simulink subsystem "tractive"  (R2023b)
settings: Solver=VariableStepAuto  StartTime=0.0  StopTime=10.0  RelTol=1e-3
libraries: Raptor_lib x11
settings Model: Creator=serga  LastModifiedBy=serga

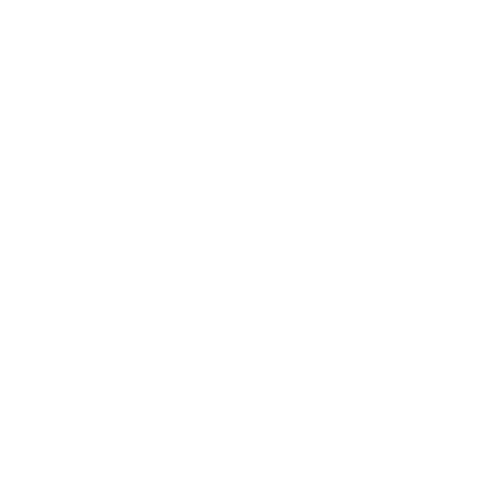
[thumbnail: Simulink's stored preview of the top-level diagram]
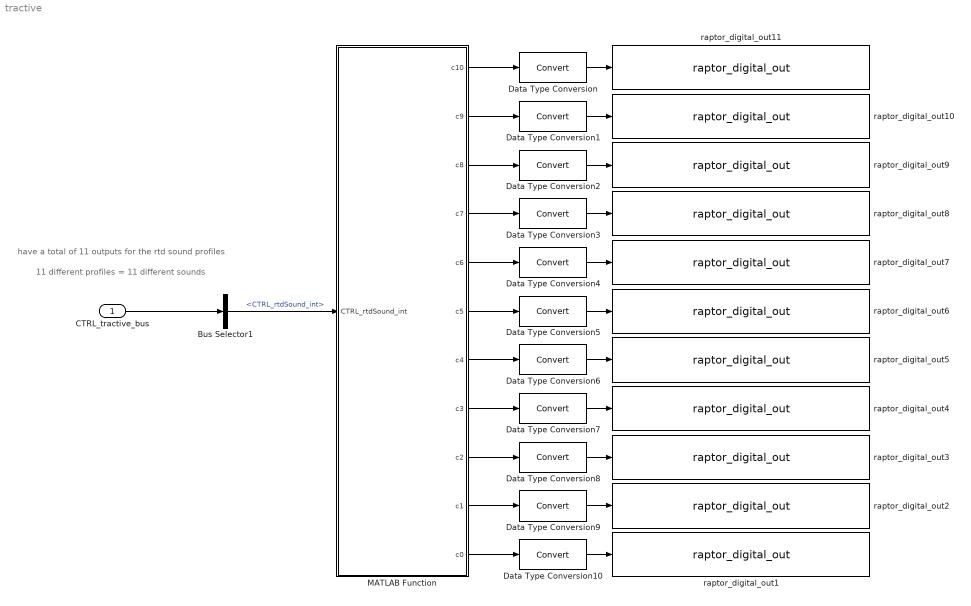
== system tractive ==
  note: 11 different profiles = 11 different sounds
  note: have a total of 11 outputs for the rtd sound profiles
  CTRL_tractive_bus : Inport
  Bus Selector1 : BusSelector  OutputSignals=CTRL_rtdSound_int
  Data Type Conversion{,1..10} (11 alike) : DataTypeConversion  SaturateOnIntegerOverflow=off  RndMeth=Floor
  MATLAB Function : MATLAB Function  TreatAsAtomicUnit=on
  raptor_digital_out1 : Raptor_lib/Input & Output/raptor_digital_out  resourceValues=OUTPUT1|OUTPUT2|OUTPUT3|OUTPUT4|OUTPUT5|OUTPUT6|OUTPUT7|OUTPUT8|OUTPUT9|OUTPUT10|OUTPUT11|OUTPUT12|OUTPUT21|OUTPUT22|OUTPUT23|OUTPUT24|OUTPUT25|OUTPUT26|OUTPUT27|OUTPUT28|OUTPUT29|OUTPUT30|OUTPUT31|OUTPUT32|OUTPUT33|OUTPUT34|OUTPUT35|OUTPUT36|OUTPUT37|OUTPUT38|OUTPUT39|OUTPUT40|OUTPUT41|OUTPUT42|OUTPUT43|OUTPUT44|OUTPUT45|OUTPUT46|OUTPUT47|OUTPUT48|OUTPUT49|POWER_HOLD|(None)  resource=OUTPUT4  driverTypeValues=Low Side  driverType=Low Side
      settings: SourceProductName=Raptor
  raptor_digital_out10 : Raptor_lib/Input & Output/raptor_digital_out  resourceValues=OUTPUT1|OUTPUT2|OUTPUT3|OUTPUT4|OUTPUT5|OUTPUT6|OUTPUT7|OUTPUT8|OUTPUT9|OUTPUT10|OUTPUT11|OUTPUT12|OUTPUT21|OUTPUT22|OUTPUT23|OUTPUT24|OUTPUT25|OUTPUT26|OUTPUT27|OUTPUT28|OUTPUT29|OUTPUT30|OUTPUT31|OUTPUT32|OUTPUT33|OUTPUT34|OUTPUT35|OUTPUT36|OUTPUT37|OUTPUT38|OUTPUT39|OUTPUT40|OUTPUT41|OUTPUT42|OUTPUT43|OUTPUT44|OUTPUT45|OUTPUT46|OUTPUT47|OUTPUT48|OUTPUT49|POWER_HOLD|(None)  resource=OUTPUT32  driverTypeValues=Low Side  driverType=Low Side
      settings: SourceProductName=Raptor
  raptor_digital_out11 : Raptor_lib/Input & Output/raptor_digital_out  resourceValues=OUTPUT1|OUTPUT2|OUTPUT3|OUTPUT4|OUTPUT5|OUTPUT6|OUTPUT7|OUTPUT8|OUTPUT9|OUTPUT10|OUTPUT11|OUTPUT12|OUTPUT21|OUTPUT22|OUTPUT23|OUTPUT24|OUTPUT25|OUTPUT26|OUTPUT27|OUTPUT28|OUTPUT29|OUTPUT30|OUTPUT31|OUTPUT32|OUTPUT33|OUTPUT34|OUTPUT35|OUTPUT36|OUTPUT37|OUTPUT38|OUTPUT39|OUTPUT40|OUTPUT41|OUTPUT42|OUTPUT43|OUTPUT44|OUTPUT45|OUTPUT46|OUTPUT47|OUTPUT48|OUTPUT49|POWER_HOLD|(None)  resource=OUTPUT35  driverTypeValues=Low Side  driverType=Low Side
      settings: SourceProductName=Raptor
  raptor_digital_out2 : Raptor_lib/Input & Output/raptor_digital_out  resourceValues=OUTPUT1|OUTPUT2|OUTPUT3|OUTPUT4|OUTPUT5|OUTPUT6|OUTPUT7|OUTPUT8|OUTPUT9|OUTPUT10|OUTPUT11|OUTPUT12|OUTPUT21|OUTPUT22|OUTPUT23|OUTPUT24|OUTPUT25|OUTPUT26|OUTPUT27|OUTPUT28|OUTPUT29|OUTPUT30|OUTPUT31|OUTPUT32|OUTPUT33|OUTPUT34|OUTPUT35|OUTPUT36|OUTPUT37|OUTPUT38|OUTPUT39|OUTPUT40|OUTPUT41|OUTPUT42|OUTPUT43|OUTPUT44|OUTPUT45|OUTPUT46|OUTPUT47|OUTPUT48|OUTPUT49|POWER_HOLD|(None)  resource=OUTPUT22  driverTypeValues=Low Side  driverType=Low Side
      settings: SourceProductName=Raptor
  raptor_digital_out3 : Raptor_lib/Input & Output/raptor_digital_out  resourceValues=OUTPUT1|OUTPUT2|OUTPUT3|OUTPUT4|OUTPUT5|OUTPUT6|OUTPUT7|OUTPUT8|OUTPUT9|OUTPUT10|OUTPUT11|OUTPUT12|OUTPUT21|OUTPUT22|OUTPUT23|OUTPUT24|OUTPUT25|OUTPUT26|OUTPUT27|OUTPUT28|OUTPUT29|OUTPUT30|OUTPUT31|OUTPUT32|OUTPUT33|OUTPUT34|OUTPUT35|OUTPUT36|OUTPUT37|OUTPUT38|OUTPUT39|OUTPUT40|OUTPUT41|OUTPUT42|OUTPUT43|OUTPUT44|OUTPUT45|OUTPUT46|OUTPUT47|OUTPUT48|OUTPUT49|POWER_HOLD|(None)  resource=OUTPUT24  driverTypeValues=Low Side  driverType=Low Side
      settings: SourceProductName=Raptor
  raptor_digital_out4 : Raptor_lib/Input & Output/raptor_digital_out  resourceValues=OUTPUT1|OUTPUT2|OUTPUT3|OUTPUT4|OUTPUT5|OUTPUT6|OUTPUT7|OUTPUT8|OUTPUT9|OUTPUT10|OUTPUT11|OUTPUT12|OUTPUT21|OUTPUT22|OUTPUT23|OUTPUT24|OUTPUT25|OUTPUT26|OUTPUT27|OUTPUT28|OUTPUT29|OUTPUT30|OUTPUT31|OUTPUT32|OUTPUT33|OUTPUT34|OUTPUT35|OUTPUT36|OUTPUT37|OUTPUT38|OUTPUT39|OUTPUT40|OUTPUT41|OUTPUT42|OUTPUT43|OUTPUT44|OUTPUT45|OUTPUT46|OUTPUT47|OUTPUT48|OUTPUT49|POWER_HOLD|(None)  resource=OUTPUT25  driverTypeValues=Low Side  driverType=Low Side
      settings: SourceProductName=Raptor
  raptor_digital_out5 : Raptor_lib/Input & Output/raptor_digital_out  resourceValues=OUTPUT1|OUTPUT2|OUTPUT3|OUTPUT4|OUTPUT5|OUTPUT6|OUTPUT7|OUTPUT8|OUTPUT9|OUTPUT10|OUTPUT11|OUTPUT12|OUTPUT21|OUTPUT22|OUTPUT23|OUTPUT24|OUTPUT25|OUTPUT26|OUTPUT27|OUTPUT28|OUTPUT29|OUTPUT30|OUTPUT31|OUTPUT32|OUTPUT33|OUTPUT34|OUTPUT35|OUTPUT36|OUTPUT37|OUTPUT38|OUTPUT39|OUTPUT40|OUTPUT41|OUTPUT42|OUTPUT43|OUTPUT44|OUTPUT45|OUTPUT46|OUTPUT47|OUTPUT48|OUTPUT49|POWER_HOLD|(None)  resource=OUTPUT26  driverTypeValues=Low Side  driverType=Low Side
      settings: SourceProductName=Raptor
  raptor_digital_out6 : Raptor_lib/Input & Output/raptor_digital_out  resourceValues=OUTPUT1|OUTPUT2|OUTPUT3|OUTPUT4|OUTPUT5|OUTPUT6|OUTPUT7|OUTPUT8|OUTPUT9|OUTPUT10|OUTPUT11|OUTPUT12|OUTPUT21|OUTPUT22|OUTPUT23|OUTPUT24|OUTPUT25|OUTPUT26|OUTPUT27|OUTPUT28|OUTPUT29|OUTPUT30|OUTPUT31|OUTPUT32|OUTPUT33|OUTPUT34|OUTPUT35|OUTPUT36|OUTPUT37|OUTPUT38|OUTPUT39|OUTPUT40|OUTPUT41|OUTPUT42|OUTPUT43|OUTPUT44|OUTPUT45|OUTPUT46|OUTPUT47|OUTPUT48|OUTPUT49|POWER_HOLD|(None)  resource=OUTPUT27  driverTypeValues=Low Side  driverType=Low Side
      settings: SourceProductName=Raptor
  raptor_digital_out7 : Raptor_lib/Input & Output/raptor_digital_out  resourceValues=OUTPUT1|OUTPUT2|OUTPUT3|OUTPUT4|OUTPUT5|OUTPUT6|OUTPUT7|OUTPUT8|OUTPUT9|OUTPUT10|OUTPUT11|OUTPUT12|OUTPUT21|OUTPUT22|OUTPUT23|OUTPUT24|OUTPUT25|OUTPUT26|OUTPUT27|OUTPUT28|OUTPUT29|OUTPUT30|OUTPUT31|OUTPUT32|OUTPUT33|OUTPUT34|OUTPUT35|OUTPUT36|OUTPUT37|OUTPUT38|OUTPUT39|OUTPUT40|OUTPUT41|OUTPUT42|OUTPUT43|OUTPUT44|OUTPUT45|OUTPUT46|OUTPUT47|OUTPUT48|OUTPUT49|POWER_HOLD|(None)  resource=OUTPUT28  driverTypeValues=Low Side  driverType=Low Side
      settings: SourceProductName=Raptor
  raptor_digital_out8 : Raptor_lib/Input & Output/raptor_digital_out  resourceValues=OUTPUT1|OUTPUT2|OUTPUT3|OUTPUT4|OUTPUT5|OUTPUT6|OUTPUT7|OUTPUT8|OUTPUT9|OUTPUT10|OUTPUT11|OUTPUT12|OUTPUT21|OUTPUT22|OUTPUT23|OUTPUT24|OUTPUT25|OUTPUT26|OUTPUT27|OUTPUT28|OUTPUT29|OUTPUT30|OUTPUT31|OUTPUT32|OUTPUT33|OUTPUT34|OUTPUT35|OUTPUT36|OUTPUT37|OUTPUT38|OUTPUT39|OUTPUT40|OUTPUT41|OUTPUT42|OUTPUT43|OUTPUT44|OUTPUT45|OUTPUT46|OUTPUT47|OUTPUT48|OUTPUT49|POWER_HOLD|(None)  resource=OUTPUT29  driverTypeValues=Low Side  driverType=Low Side
      settings: SourceProductName=Raptor
  raptor_digital_out9 : Raptor_lib/Input & Output/raptor_digital_out  resourceValues=OUTPUT1|OUTPUT2|OUTPUT3|OUTPUT4|OUTPUT5|OUTPUT6|OUTPUT7|OUTPUT8|OUTPUT9|OUTPUT10|OUTPUT11|OUTPUT12|OUTPUT21|OUTPUT22|OUTPUT23|OUTPUT24|OUTPUT25|OUTPUT26|OUTPUT27|OUTPUT28|OUTPUT29|OUTPUT30|OUTPUT31|OUTPUT32|OUTPUT33|OUTPUT34|OUTPUT35|OUTPUT36|OUTPUT37|OUTPUT38|OUTPUT39|OUTPUT40|OUTPUT41|OUTPUT42|OUTPUT43|OUTPUT44|OUTPUT45|OUTPUT46|OUTPUT47|OUTPUT48|OUTPUT49|POWER_HOLD|(None)  resource=OUTPUT30  driverTypeValues=Low Side  driverType=Low Side
      settings: SourceProductName=Raptor
  wires:
  CTRL_tractive_bus/1 -> Bus Selector1/1
  Bus Selector1/1 -> MATLAB Function/1(CTRL_rtdSound_int)  "<CTRL_rtdSound_int>"
  MATLAB Function/11(c0) -> Data Type Conversion10/1
  MATLAB Function/1(c10) -> Data Type Conversion/1
  MATLAB Function/2(c9) -> Data Type Conversion1/1
  MATLAB Function/3(c8) -> Data Type Conversion2/1
  MATLAB Function/4(c7) -> Data Type Conversion3/1
  MATLAB Function/6(c5) -> Data Type Conversion5/1
  MATLAB Function/5(c6) -> Data Type Conversion4/1
  MATLAB Function/7(c4) -> Data Type Conversion6/1
  MATLAB Function/8(c3) -> Data Type Conversion7/1
  MATLAB Function/9(c2) -> Data Type Conversion8/1
  MATLAB Function/10(c1) -> Data Type Conversion9/1
  Data Type Conversion/1 -> raptor_digital_out11/1
  Data Type Conversion1/1 -> raptor_digital_out10/1
  Data Type Conversion2/1 -> raptor_digital_out9/1
  Data Type Conversion3/1 -> raptor_digital_out8/1
  Data Type Conversion4/1 -> raptor_digital_out7/1
  Data Type Conversion5/1 -> raptor_digital_out6/1
  Data Type Conversion6/1 -> raptor_digital_out5/1
  Data Type Conversion7/1 -> raptor_digital_out4/1
  Data Type Conversion8/1 -> raptor_digital_out3/1
  Data Type Conversion9/1 -> raptor_digital_out2/1
  Data Type Conversion10/1 -> raptor_digital_out1/1

== matlab function tractive/MATLAB Function ==
  data: CTRL_rtdSound_int input; c10 output; c9 output; c8 output; c7 output; c6 output; c5 output; c4 output; c3 output; c2 output; c1 output; c0 output
function [c10,c9,c8,c7,c6,c5,c4,c3,c2,c1,c0] = fcn(CTRL_rtdSound_int)

if CTRL_rtdSound_int == 10
    c10 = 1; c9 = 0; c8 = 0; c7 = 0; c6 = 0; c5 = 0; c4 = 0; c3 = 0; c2 = 0; c1 = 0; c0 = 0;
elseif CTRL_rtdSound_int == 9
    c10 = 0; c9 = 1; c8 = 0; c7 = 0; c6 = 0; c5 = 0; c4 = 0; c3 = 0; c2 = 0; c1 = 0; c0 = 0;
elseif CTRL_rtdSound_int == 8
    c10 = 0; c9 = 0; c8 = 1; c7 = 0; c6 = 0; c5 = 0; c4 = 0; c3 = 0; c2 = 0; c1 = 0; c0 = 0;
elseif CTRL_rtdSound_int == 7
    c10 = 0; c9 = 0; c8 = 0; c7 = 1; c6 = 0; c5 = 0; c4 = 0; c3 = 0; c2 = 0; c1 = 0; c0 = 0;
elseif CTRL_rtdSound_int == 6
    c10 = 0; c9 = 0; c8 = 0; c7 = 0; c6 = 1; c5 = 0; c4 = 0; c3 = 0; c2 = 0; c1 = 0; c0 = 0;
elseif CTRL_rtdSound_int == 5
    c10 = 0; c9 = 0; c8 = 0; c7 = 0; c6 = 0; c5 = 1; c4 = 0; c3 = 0; c2 = 0; c1 = 0; c0 = 0;
elseif CTRL_rtdSound_int == 4
    c10 = 0; c9 = 0; c8 = 0; c7 = 0; c6 = 0; c5 = 0; c4 = 1; c3 = 0; c2 = 0; c1 = 0; c0 = 0;
elseif CTRL_rtdSound_int == 3
    c10 = 0; c9 = 0; c8 = 0; c7 = 0; c6 = 0; c5 = 0; c4 = 0; c3 = 1; c2 = 0; c1 = 0; c0 = 0;
elseif CTRL_rtdSound_int == 2
    c10 = 0; c9 = 0; c8 = 0; c7 = 0; c6 = 0; c5 = 0; c4 = 0; c3 = 0; c2 = 1; c1 = 0; c0 = 0;
elseif CTRL_rtdSound_int == 1
    c10 = 0; c9 = 0; c8 = 0; c7 = 0; c6 = 0; c5 = 0; c4 = 0; c3 = 0; c2 = 0; c1 = 1; c0 = 0;
else
    c10 = 0; c9 = 0; c8 = 0; c7 = 0; c6 = 0; c5 = 0; c4 = 0; c3 = 0; c2 = 0; c1 = 0; c0 = 1;
end
